simulink model "FCEvReferenceApplication"  (R2023a)
settings: Solver=ode23t  StartTime=0  StopTime=1435  RelTol=1e-3  EnableMultiTasking=on
libraries: autolibshared x1
settings Model: DataDictionary=VehicleConfig.sldd  ModifiedByFormat=The MathWorks, Inc.  SimulationMode=accelerator  PauseTimes=0  Creator=The MathWorks, Inc.  LastModifiedBy=The MathWorks, Inc.
settings SolverCC: MaxConsecutiveMinStep=12  ZeroCrossAlgorithm=Adaptive  AlgebraicLoopSolver=TrustRegion  AutoInsertRateTranBlk=on  DecoupledContinuousIntegration=on  MinimalZcImpactIntegration=on  MaxZcPerStep=1
settings DataIOCC: SaveOutput=off  DSMLogging=off  SaveTime=off  ReturnWorkspaceOutputs=off
settings OptimizationCC: ReuseModelBlockBuffer=off
settings DebuggingCC: UnderspecifiedInitializationDetection=Classic  MergeDetectMultiDrivingBlocksExec=none  IgnoredZcDiagnostic=none  UnconnectedInputMsg=warning  UnconnectedOutputMsg=warning  UnconnectedLineMsg=warning  ModelReferenceExtraNoncontSigs=none  PregeneratedLibrarySubsystemCodeDiagnostic=none  ArithmeticOperatorsInVariantConditions=warning
settings ModelReferenceCC: UpdateModelReferenceTargets=IfOutOfDate  EnableRefExpFcnMdlSchedulingChecks=on  ModelReferenceMinAlgLoopOccurrences=on  PropagateSignalLabelsOutOfModel=off
settings SFSimCC: SimUseLocalCustomCode=off
settings RTWCC: RTWUseLocalCustomCode=off  Toolchain=Microsoft Visual C++ 2022 v17.0 | CMake/nmake (64-bit Windows)  BuildConfiguration=Release  DLArmComputeVersion=19.05
settings CodeAppCC: StateflowObjectComments=on
settings GRTTargetCC: TargetLangStandard=C89/C90 (ANSI)
settings ConfigComp: CovMetricSettings=dsw  CovSaveCumulativeToWorkspaceVar=on  CovSaveSingleToWorkspaceVar=on  CovExternalEMLEnable=off

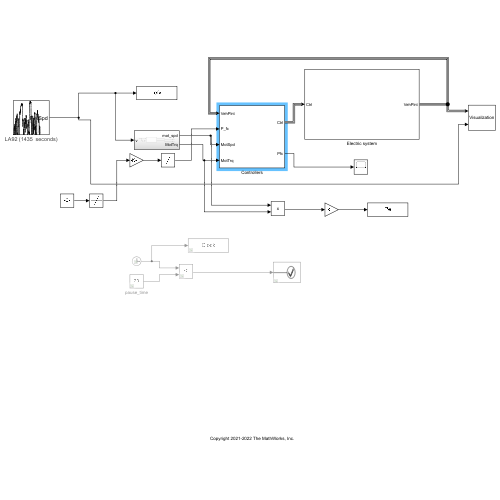
[thumbnail: Simulink's stored preview of the top-level diagram]
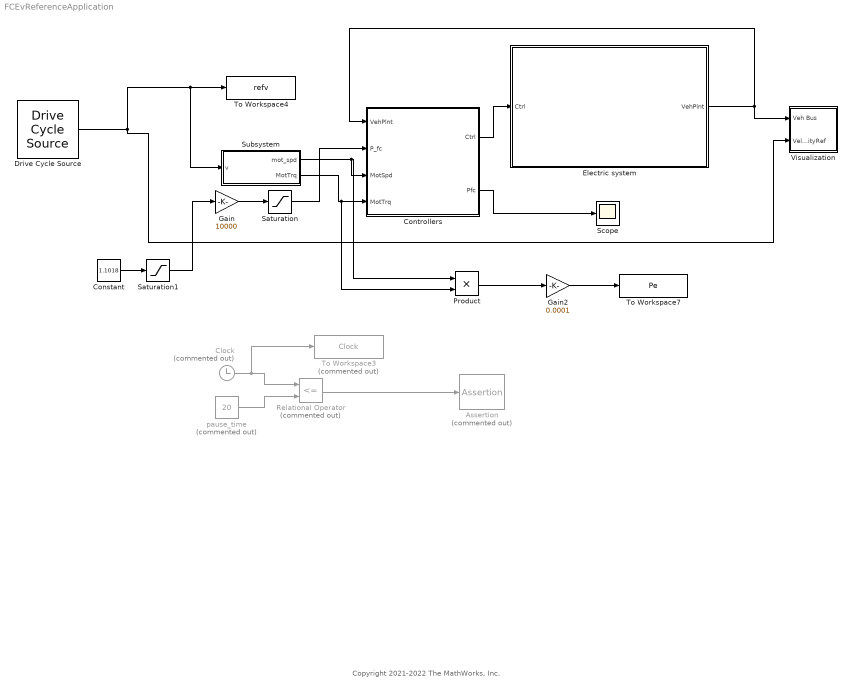
== system FCEvReferenceApplication ==
  note: Copyright 2021-2022 The MathWorks, Inc.
  Assertion : Assertion  Commented=on  AssertionFailFcn=set_param(bdroot, 'SimulationCommand', 'pause')  StopWhenAssertionFail=off
  Clock : Clock  Commented=on
  Constant : Constant  Value=1.1018
  Controllers : Subsystem
  Drive Cycle Source : autolibshared/Drive Cycle Source  cycleVar=LA92  fileVar=C:\Users\Leviathan\Desktop\WLTC工况.xlsx  tfinal="1435  seconds"  cycleRepeat=off  outAccPort=off  outGearPort=off  gearList=No gear data  t_wot1=1  xdot_woto=0  xdot_wot1=26.8  t_wot2=30  xdot_wot2=0  t_wotend=40  srcUnit=m/s  outUnit=m/s  srcAccUnit=m/s/s  outAccUnit=m/s^2  dt=0  aMode=1  faultOption=off  velBnd=2  velBndUnit=mph  inUnit=m/s  timeBnd=1  failOption=off  stopSim=off  maxFaultCnt=10  maxFaultTime=2  maxTotFaultTime=15  traceOption=off  dtTrace=1  traceWindow=10  lastDCname=LA92  lastOutUnit=mph  lastDT=0  lastTB=1  lastSB=2  forceCalcBound=off
  Electric system : Subsystem
  Gain : Gain  Gain=10000
  Gain2 : Gain  Gain=0.0001
  Product : Product
  Relational Operator : RelationalOperator  Commented=on  Operator=<=  OutDataTypeStr=boolean  RndMeth=Simplest  InputSameDT=off
  Saturation : Saturate  UpperLimit=inf  LowerLimit=200
  Saturation1 : Saturate  UpperLimit=35  LowerLimit=0
  Scope : Scope
  Subsystem : Subsystem
  To Workspace3 : ToWorkspace  Commented=on  VariableName=Clock  SampleTime=1
  To Workspace4 : ToWorkspace  VariableName=refv  SampleTime=1
  To Workspace7 : ToWorkspace  VariableName=Pe  SampleTime=1
  Visualization : Subsystem
      mask Display: disp(getString(message('autoblks:autoblkVehMask:visual')))
  pause_time : Constant  Commented=on  Value=20
  wires:
  Controllers/1(Ctrl) -> Electric system/1(Ctrl)
  Electric system/1(VehPlnt) -> Visualization/1(Veh Bus), Controllers/1(VehPlnt)
  Controllers/2(Pfc) -> Scope/1
  pause_time/1 -> Relational Operator/2
  Clock/1 -> To Workspace3/1, Relational Operator/1
  Relational Operator/1 -> Assertion/1
  Gain/1 -> Saturation/1
  Constant/1 -> Saturation1/1
  Saturation1/1 -> Gain/1
  Subsystem/1(mot_spd) -> Product/1, Controllers/3(MotSpd)
  Subsystem/2(MotTrq) -> Product/2, Controllers/4(MotTrq)
  Drive Cycle Source/1 -> Visualization/2(VelocityRef), Subsystem/1(v), To Workspace4/1
  Gain2/1 -> To Workspace7/1
  Product/1 -> Gain2/1
  Saturation/1 -> Controllers/2(P_fc)

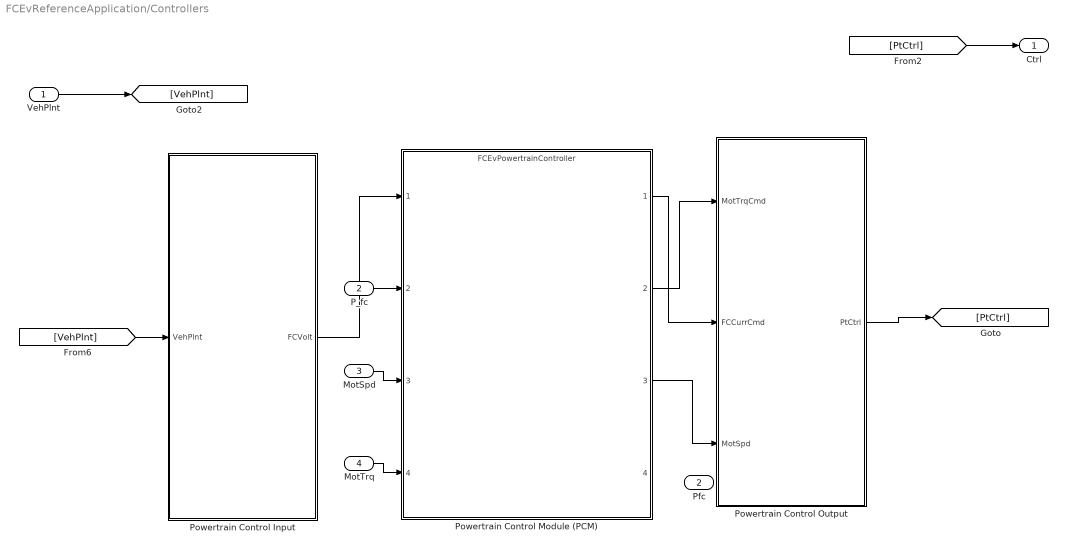
== system FCEvReferenceApplication/Controllers ==
  VehPlnt : Inport
  P_fc : Inport  Port=2
  MotSpd : Inport  Port=3
  MotTrq : Inport  Port=4
  Powertrain Control Input : Subsystem
  Powertrain Control Module (PCM) : ModelReference  ModelNameDialog=FCEvPowertrainController.slx  ModelReferenceVersion=6.39
  Powertrain Control Output : Subsystem
  Ctrl : Outport  VectorParamsAs1DForOutWhenUnconnected=off
  Pfc : Outport  Port=2
  wires:
  VehPlnt/1 -> [VehPlnt]
  [PtCtrl] -> Ctrl/1
  [VehPlnt] -> Powertrain Control Input/1(VehPlnt)
  Powertrain Control Output/1(PtCtrl) -> [PtCtrl]
  Powertrain Control Input/1(FCVolt) -> Powertrain Control Module (PCM)/1
  Powertrain Control Module (PCM)/1 -> Powertrain Control Output/2(FCCurrCmd)
  Powertrain Control Module (PCM)/3 -> Powertrain Control Output/3(MotSpd)
  MotTrq/1 -> Powertrain Control Module (PCM)/4
  MotSpd/1 -> Powertrain Control Module (PCM)/3
  Powertrain Control Module (PCM)/2 -> Powertrain Control Output/1(MotTrqCmd)
  P_fc/1 -> Powertrain Control Module (PCM)/2
  ? -> Pfc/1

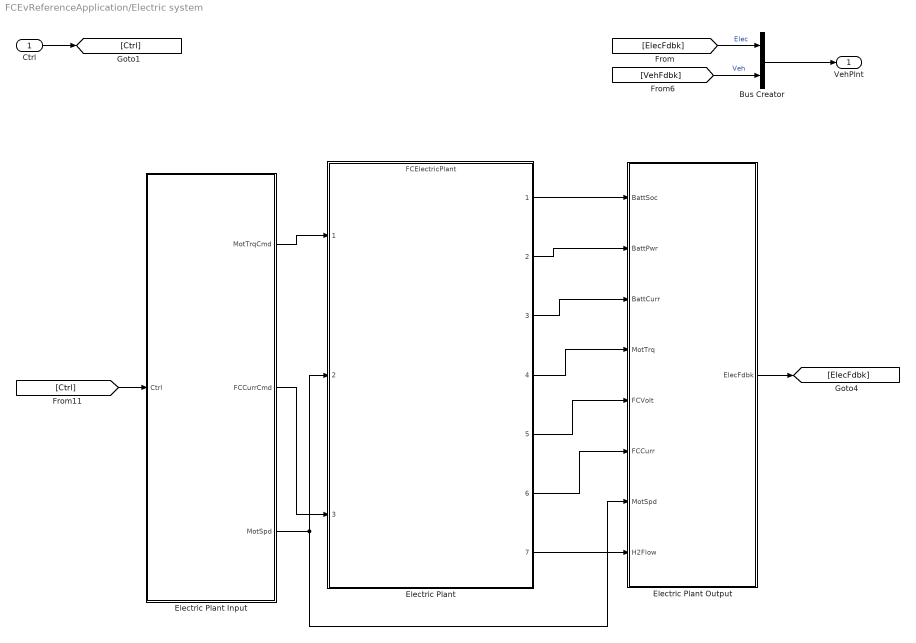
== system FCEvReferenceApplication/Electric system ==
  Ctrl : Inport
  Bus Creator : BusCreator  Inputs=2
  Electric Plant : ModelReference  ModelNameDialog=FCElectricPlant.slx  ModelReferenceVersion=6.24
  Electric Plant Input : Subsystem
  Electric Plant Output : Subsystem
  VehPlnt : Outport  VectorParamsAs1DForOutWhenUnconnected=off
  wires:
  Electric Plant/1 -> Electric Plant Output/1(BattSoc)
  Electric Plant/6 -> Electric Plant Output/6(FCCurr)
  Electric Plant/5 -> Electric Plant Output/5(FCVolt)
  Electric Plant/3 -> Electric Plant Output/3(BattCurr)
  Electric Plant/4 -> Electric Plant Output/4(MotTrq)
  Bus Creator/1 -> VehPlnt/1
  [ElecFdbk] -> Bus Creator/1  "Elec"
  Electric Plant Output/1(ElecFdbk) -> [ElecFdbk]
  Electric Plant Input/1(MotTrqCmd) -> Electric Plant/1
  Electric Plant/2 -> Electric Plant Output/2(BattPwr)
  [VehFdbk] -> Bus Creator/2  "Veh"
  [Ctrl] -> Electric Plant Input/1(Ctrl)
  Ctrl/1 -> [Ctrl]
  Electric Plant Input/2(FCCurrCmd) -> Electric Plant/3
  Electric Plant Input/3(MotSpd) -> Electric Plant Output/7(MotSpd), Electric Plant/2
  Electric Plant/7 -> Electric Plant Output/8(H2Flow)

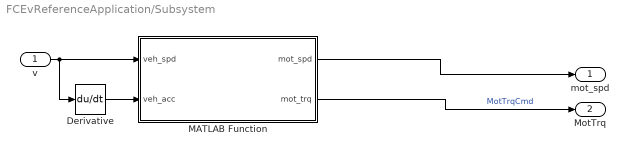
== system FCEvReferenceApplication/Subsystem ==
  v : Inport
  Derivative : Derivative
  MATLAB Function : MATLAB Function  TreatAsAtomicUnit=on
  mot_spd : Outport
  MotTrq : Outport  Port=2
  wires:
  v/1 -> Derivative/1, MATLAB Function/1(veh_spd)
  MATLAB Function/1(mot_spd) -> mot_spd/1
  MATLAB Function/2(mot_trq) -> MotTrq/1  "MotTrqCmd"
  Derivative/1 -> MATLAB Function/2(veh_acc)

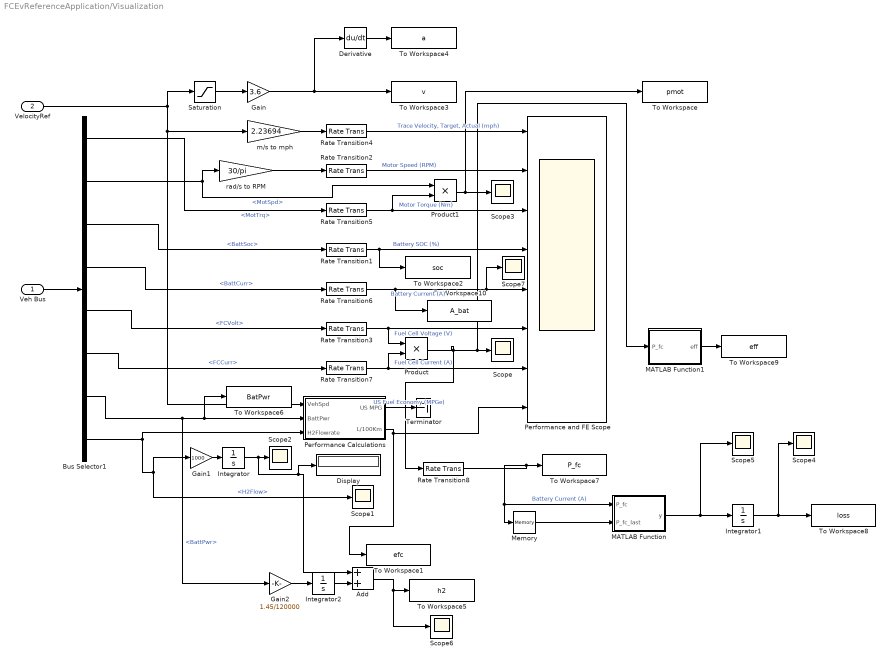
== system FCEvReferenceApplication/Visualization ==
  Veh Bus : Inport
  VelocityRef : Inport  Port=2
  Add : Sum
  Bus Selector1 : BusSelector  OutputSignals=Elec.MotTrq,Elec.MotSpd,Elec.BattSoc,Elec.BattCurr,Elec.FCVolt,Elec.FCCurr,Elec.BattPwr,Elec.H2Flow
  Derivative : Derivative
  Display : Display
  Gain : Gain  Gain=3.6
  Gain1 : Gain  Gain=1000
  Gain2 : Gain  Gain=1.45/120000
  Integrator : Integrator
  Integrator1 : Integrator
  Integrator2 : Integrator
  MATLAB Function : MATLAB Function  TreatAsAtomicUnit=on
  MATLAB Function1 : MATLAB Function  TreatAsAtomicUnit=on
  Memory : Memory  InheritSampleTime=on
  Performance Calculations : Subsystem
  Performance and FE Scope : Scope  NumInputPorts=8
  Product : Product
  Product1 : Product
  Rate Transition{1..2,4..6} (5 alike) : RateTransition  Deterministic=off
  Rate Transition3 : RateTransition  Deterministic=off  OutPortSampleTime=1
  Rate Transition7 : RateTransition  Deterministic=off  OutPortSampleTime=1
  Rate Transition8 : RateTransition  Deterministic=off  OutPortSampleTime=1
  Saturation : Saturate  UpperLimit=Inf  LowerLimit=0
  Scope{,1..7} (8 alike) : Scope
  Terminator : Terminator
  To Workspace : ToWorkspace  VariableName=pmot  SampleTime=1
  To Workspace1 : ToWorkspace  VariableName=efc  SampleTime=1
  To Workspace10 : ToWorkspace  VariableName=A_bat  SampleTime=1
  To Workspace2 : ToWorkspace  VariableName=soc  SampleTime=1
      settings: Save2DSignal=2-D array (concatenate along first dimension)
  To Workspace3 : ToWorkspace  VariableName=v  SampleTime=1
  To Workspace4 : ToWorkspace  VariableName=a  SampleTime=1
  To Workspace5 : ToWorkspace  VariableName=h2  SampleTime=1
  To Workspace6 : ToWorkspace  VariableName=BatPwr  SampleTime=1
      settings: Save2DSignal=2-D array (concatenate along first dimension)
  To Workspace7 : ToWorkspace  VariableName=P_fc  SampleTime=1
  To Workspace8 : ToWorkspace  VariableName=loss  SampleTime=1
  To Workspace9 : ToWorkspace  VariableName=eff  SampleTime=1
  m/s to mph : Gain  Gain=2.23694
  rad/s to RPM : Gain  Gain=30/pi
  wires:
  Veh Bus/1 -> Bus Selector1/1
  VelocityRef/1 -> Performance Calculations/1(VehSpd), m/s to mph/1, Saturation/1
  Performance Calculations/2(L/100Km) -> Performance and FE Scope/8, To Workspace1/1
  m/s to mph/1 -> Rate Transition4/1
  Bus Selector1/3 -> Rate Transition1/1  "<BattSoc>"
  Rate Transition1/1 -> To Workspace2/1, Performance and FE Scope/4  "Battery SOC (%)"
  Rate Transition2/1 -> Performance and FE Scope/2  "Motor Speed (RPM)"
  Rate Transition4/1 -> Performance and FE Scope/1  "Trace Velocity, Target, Actual (mph)"
  Bus Selector1/2 -> rad/s to RPM/1, Product1/1  "<MotSpd>"
  Bus Selector1/7 -> Gain2/1, Performance Calculations/2(BattPwr), To Workspace6/1  "<BattPwr>"
  rad/s to RPM/1 -> Rate Transition2/1
  Bus Selector1/1 -> Rate Transition5/1  "<MotTrq>"
  Rate Transition5/1 -> Product1/2, Performance and FE Scope/3  "Motor Torque (Nm)"
  Rate Transition6/1 -> To Workspace10/1, Scope7/1, Performance and FE Scope/5  "Battery Current (A)"
  Bus Selector1/4 -> Rate Transition6/1  "<BattCurr>"
  Bus Selector1/8 -> Performance Calculations/3(H2Flowrate), Scope1/1, Gain1/1  "<H2Flow>"
  Bus Selector1/6 -> Rate Transition7/1  "<FCCurr>"
  Rate Transition7/1 -> Performance and FE Scope/7, Product/2  "Fuel Cell Current (A)"
  Bus Selector1/5 -> Rate Transition3/1  "<FCVolt>"
  Rate Transition3/1 -> Performance and FE Scope/6, Product/1  "Fuel Cell Voltage (V)"
  Product/1 -> Rate Transition8/1, MATLAB Function1/1(P_fc), Scope/1
  Saturation/1 -> Gain/1
  Gain/1 -> Derivative/1, To Workspace3/1
  Derivative/1 -> To Workspace4/1
  Integrator/1 -> Add/1, Display/1, Scope2/1
  Gain1/1 -> Integrator/1
  Performance Calculations/1(US MPG) -> Terminator/1  "US Fuel Economy (MPGe)"
  Product1/1 -> To Workspace/1, Scope3/1
  Memory/1 -> MATLAB Function/2(P_fc_last)
  MATLAB Function/1(y) -> Scope5/1, Integrator1/1
  Integrator1/1 -> Scope4/1, To Workspace8/1
  Gain2/1 -> Integrator2/1
  Add/1 -> Scope6/1, To Workspace5/1
  Integrator2/1 -> Add/2
  MATLAB Function1/1(eff) -> To Workspace9/1
  Rate Transition8/1 -> Memory/1, MATLAB Function/1(P_fc), To Workspace7/1  "Battery Current (A)"

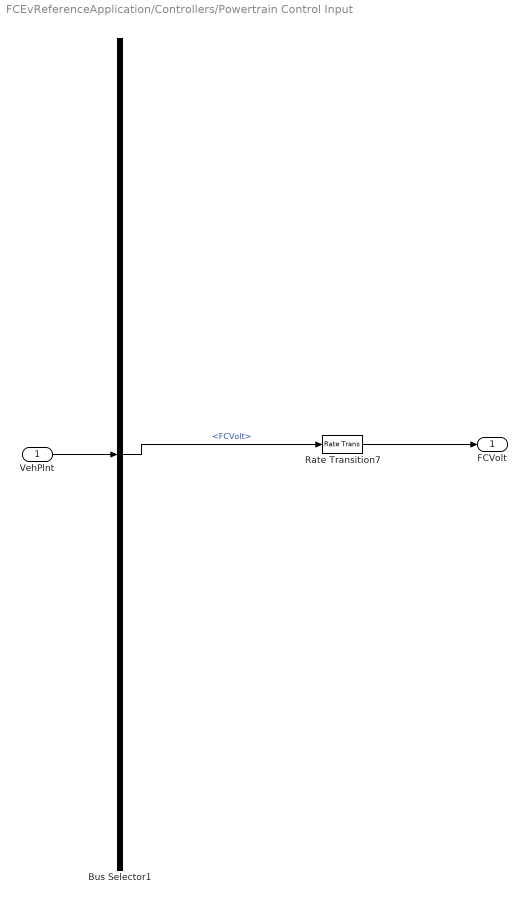
== system FCEvReferenceApplication/Controllers/Powertrain Control Input ==
  VehPlnt : Inport
  Bus Selector1 : BusSelector  OutputSignals=Elec.FCVolt
  Rate Transition7 : RateTransition  Deterministic=off
  FCVolt : Outport  VectorParamsAs1DForOutWhenUnconnected=off
  wires:
  VehPlnt/1 -> Bus Selector1/1
  Rate Transition7/1 -> FCVolt/1
  Bus Selector1/1 -> Rate Transition7/1  "<FCVolt>"

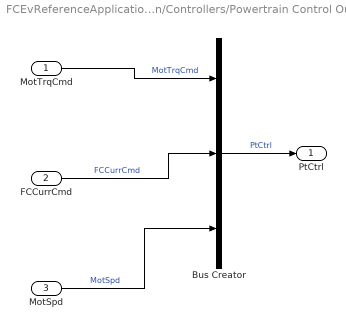
== system FCEvReferenceApplication/Controllers/Powertrain Control Output ==
  MotTrqCmd : Inport
  FCCurrCmd : Inport  Port=2
  MotSpd : Inport  Port=3
  Bus Creator : BusCreator  Inputs=3
  PtCtrl : Outport  VectorParamsAs1DForOutWhenUnconnected=off
  wires:
  Bus Creator/1 -> PtCtrl/1  "PtCtrl"
  MotTrqCmd/1 -> Bus Creator/1  "MotTrqCmd"
  FCCurrCmd/1 -> Bus Creator/2  "FCCurrCmd"
  MotSpd/1 -> Bus Creator/3  "MotSpd"

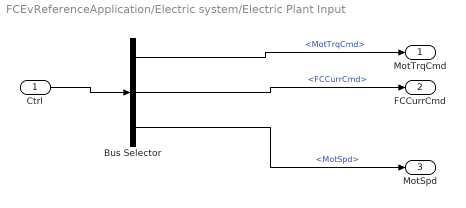
== system FCEvReferenceApplication/Electric system/Electric Plant Input ==
  Ctrl : Inport
  Bus Selector : BusSelector  OutputSignals=MotTrqCmd,FCCurrCmd,MotSpd
  MotTrqCmd : Outport  VectorParamsAs1DForOutWhenUnconnected=off
  FCCurrCmd : Outport  Port=2  VectorParamsAs1DForOutWhenUnconnected=off
  MotSpd : Outport  Port=3  VectorParamsAs1DForOutWhenUnconnected=off
  wires:
  Ctrl/1 -> Bus Selector/1
  Bus Selector/1 -> MotTrqCmd/1  "<MotTrqCmd>"
  Bus Selector/2 -> FCCurrCmd/1  "<FCCurrCmd>"
  Bus Selector/3 -> MotSpd/1  "<MotSpd>"

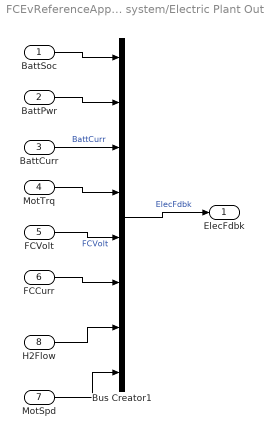
== system FCEvReferenceApplication/Electric system/Electric Plant Output ==
  BattSoc : Inport
  BattPwr : Inport  Port=2
  BattCurr : Inport  Port=3
  MotTrq : Inport  Port=4
  FCVolt : Inport  Port=5
  FCCurr : Inport  Port=6
  MotSpd : Inport  Port=7
  H2Flow : Inport  Port=8
  Bus Creator1 : BusCreator  Inputs=8
  ElecFdbk : Outport  VectorParamsAs1DForOutWhenUnconnected=off
  wires:
  Bus Creator1/1 -> ElecFdbk/1  "ElecFdbk"
  BattPwr/1 -> Bus Creator1/2
  BattSoc/1 -> Bus Creator1/1
  BattCurr/1 -> Bus Creator1/3  "BattCurr"
  MotTrq/1 -> Bus Creator1/4
  FCVolt/1 -> Bus Creator1/5  "FCVolt"
  FCCurr/1 -> Bus Creator1/6
  H2Flow/1 -> Bus Creator1/7
  MotSpd/1 -> Bus Creator1/8

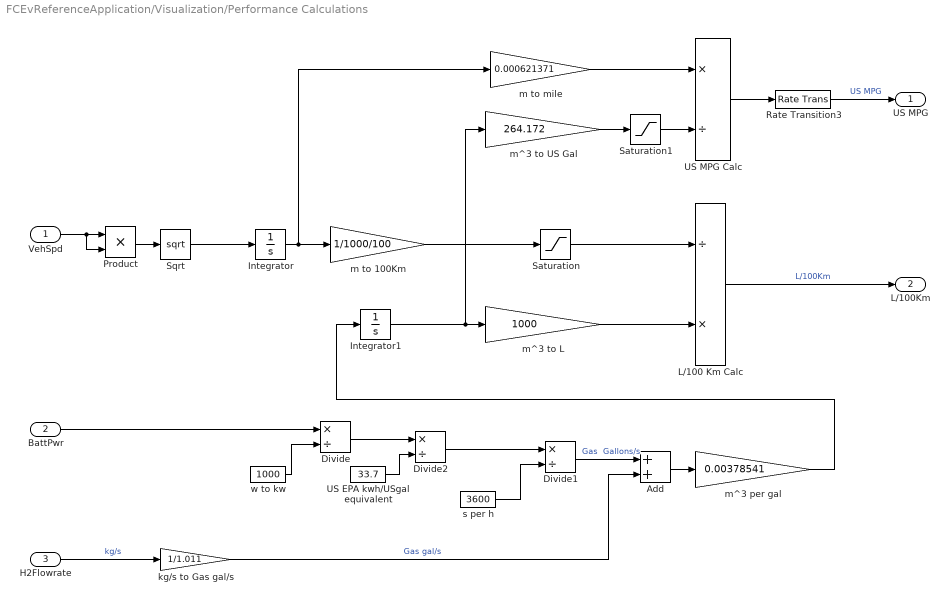
== system FCEvReferenceApplication/Visualization/Performance Calculations ==
  VehSpd : Inport
  BattPwr : Inport  Port=2
  H2Flowrate : Inport  Port=3
  Add : Sum
  Divide : Product  Inputs=*/
  Divide1 : Product  Inputs=*/
  Divide2 : Product  Inputs=*/
  Integrator : Integrator
  Integrator1 : Integrator
  L/100 Km Calc : Product  Inputs=/*
  Product : Product
  Rate Transition3 : RateTransition  Deterministic=off
  Saturation : Saturate  UpperLimit=Inf  LowerLimit=0.001
  Saturation1 : Saturate  UpperLimit=Inf  LowerLimit=1e-3
  Sqrt : Sqrt
  US EPA kwh/USgal equivalent : Constant  Value=33.7
  US MPG Calc : Product  Inputs=*/
  kg/s to Gas gal/s : Gain  Gain=1/1.011
  m to 100Km : Gain  Gain=1/1000/100
  m to mile : Gain  Gain=0.000621371
  m^3 per gal : Gain  Gain=0.00378541
  m^3 to L : Gain  Gain=1000
  m^3 to US Gal : Gain  Gain=264.172
  s per h : Constant  Value=3600
  w to kw : Constant  Value=1000
  US MPG : Outport  VectorParamsAs1DForOutWhenUnconnected=off
  L/100Km : Outport  Port=2  VectorParamsAs1DForOutWhenUnconnected=off
  wires:
  m^3 to US Gal/1 -> Saturation1/1
  m^3 to L/1 -> L/100 Km Calc/2
  Integrator/1 -> m to mile/1, m to 100Km/1
  m to mile/1 -> US MPG Calc/1
  Integrator1/1 -> m^3 to US Gal/1, m^3 to L/1
  Saturation/1 -> L/100 Km Calc/1
  m to 100Km/1 -> Saturation/1
  L/100 Km Calc/1 -> L/100Km/1  "L/100Km"
  US MPG Calc/1 -> Rate Transition3/1
  Saturation1/1 -> US MPG Calc/2
  Rate Transition3/1 -> US MPG/1  "US MPG"
  w to kw/1 -> Divide/2
  Divide/1 -> Divide2/1
  Divide2/1 -> Divide1/1
  s per h/1 -> Divide1/2
  Divide1/1 -> Add/1  "Gas  Gallons/s"
  US EPA kwh/USgal equivalent/1 -> Divide2/2
  BattPwr/1 -> Divide/1
  Sqrt/1 -> Integrator/1
  Product/1 -> Sqrt/1
  VehSpd/1 -> Product/2, Product/1
  m^3 per gal/1 -> Integrator1/1
  H2Flowrate/1 -> kg/s to Gas gal/s/1  "kg/s"
  kg/s to Gas gal/s/1 -> Add/2  "Gas gal/s"
  Add/1 -> m^3 per gal/1

== matlab function FCEvReferenceApplication/Visualization/MATLAB Function ==
  data: P_fc input; y output; P_fc_last input
function y = fcn(P_fc, P_fc_last)
u=0;
if((P_fc==0&&P_fc_last>0))
    u=u+0.00196;
end
if(P_fc>0&&P_fc<=7000)
    u=u+0.00126/3600;
end
if(abs(P_fc-P_fc_last)>12000) 
    u=u+0.00005963;
end
if(P_fc>63000)
    u=u+0.00147/3600;
end

y = u;

== matlab function FCEvReferenceApplication/Visualization/MATLAB Function1 ==
  data: P_fc input; eff output
function eff = fcn(P_fc)
fc_pwr_map = [0	1072.90229853803	1216.85650798951	1359.59851460102	1501.35017957354	1642.27676444055	1782.53778025993	1922.24351589635	2061.42626733138	2200.07476094921	2338.17130192102	2475.70683694821	2612.68288708918	2749.10918467404	2885.00072139605	3020.37535249597	3155.25212611030	3289.65020692397	3423.58823588020	3557.08391827318	3690.15380512072	3823.07558594165	3955.85245344655	4088.37561795968	4220.61488906977	4352.56406363307	4484.22506138967	4615.60845349907	4746.72537153320	4877.58617634250	5008.20101841421	5138.57910701179	5268.72893779909	5398.65843210451	5528.37491810699	5657.88512121010	5787.19531790160	5916.31126144911	6045.23838229580	6173.98170377466	6302.54592100281	6430.93523576898	6559.15407939906	6686.36322605221	6812.91227829557	6939.23197241272	7065.32770458568	7191.20233240135	7316.85868136767	7442.29946015133	7567.52735310215	7692.54476785426	7817.35414262247	7941.95794027495	8066.35839410929	8190.55721576634	8314.55761866446	8438.36117790742	8561.96941744725	8685.38463779521	8808.60863685525	8931.64323689573	9054.49014325740	9177.15069874731	9299.62695433075	9421.92021588226	9544.03195449078	9665.96362107524	9787.71705237388	9909.29339377050	10030.6937637603	10151.9199164870	10272.9726013835	10393.8537048637	10514.5636761990	10635.1045530165	10755.4772713985	10875.6826157159	10995.7216879776	11115.5959476105	11235.3059832979	11354.8530825862	11474.2382729129	11593.4622572804	11712.5261226507	11831.4307634265	11950.1772445910	12068.7664326711	12187.1991631663	12305.4762984413	12423.5986606479	12541.5671462540	12659.3824194685	12777.0451010561	12894.5559678070	13011.9203853400	13129.1509406938	13246.2534270434	13363.2291458499	13480.0764252504	13596.7929126851	13713.3756818561	13829.8227998316	13946.1318121346	14062.3022020181	14178.3328702196	14294.2229916514	14409.9724360912	14525.5811090914	14641.0491037678	14756.3766437677	14871.5640268236	14986.6116165973	15101.5198142293	15216.2890283615	15330.9196985154	15445.4122669574	15559.7671786892	15673.9848782481	15788.0658123241	15902.0104005133	16015.8190981300	16129.4923319684	16243.0305028681	16356.4340315659	16469.7033383789	16582.8388327729	16695.8408921659	16808.7099143940	16921.4462843248	17034.0503807289	17146.5225766003	17258.8632395181	17371.0727307757	17483.1514069888	17595.0996192849	17706.9177135773	17818.6060306982	17930.1649065130	18041.5946720314	18152.8956534897	18264.0681724165	18375.1125459202	18486.0290866848	18596.8181030627	18707.4798991736	18818.0147750123	18928.4230265502	19038.7049458338	19148.8608210861	19258.8909368034	19368.7955738538	19478.5750095701	19588.2295178478	19697.7593692369	19807.1648310362	19916.4461673844	20025.6036393511	20134.6375050283	20243.5480196198	20352.3354355281	20461.0000024441	20569.5419583178	20677.9613366887	20786.2582763735	20894.4329891170	21002.4856857775	21110.4165737466	21218.2258576406	21325.9137386505	21433.4804149482	21540.9260816950	21648.2509310959	21755.4551524525	21862.5389322177	21969.5024540466	22076.3458988475	22183.0694448317	22289.6732675625	22396.1575400017	22502.5224325584	22608.7681131334	22714.8947471644	22820.9024976699	22926.7915255296	23032.5619885719	23138.2140430316	23243.7478426889	23349.1635390930	23454.4612816159	23559.6412174922	23664.7034918522	23769.6482477691	23874.4756262756	23979.1857662239	24083.7788051244	24188.2548782964	24292.6141177574	24396.8566560881	24500.9826225012	24604.9921447184	24708.8853487057	24812.6623586889	24916.3232971743	25019.8682849774	25123.2974412481	25226.6108834969	25329.8087283243	25432.8910951689	25535.8580953686	25638.7098392918	25741.4464360553	25844.0679934139	25946.5746177226	26048.9664139350	26151.2434856103	26253.4059349319	26355.4538627218	26457.3873684589	26559.2065502960	26660.9115050783	26762.5023283583	26863.9791144160	26965.3419562732	27066.5909457112	27167.7261732871	27268.7477283497	27369.6556988230	27470.4501724288	27571.1312344540	27671.6989694970	27772.1534609557	27872.4947914538	27972.7230415141	28072.8382934268	28172.8406249958	28272.7301143478	28372.5068379005	28472.1708730543	28571.7222948795	28671.1611756256	28770.4875900029	28869.7016088879	28968.8033038351	29067.7927456532	29166.6700009573	29265.4351410368	29364.0882311638	29462.6293378617	29561.0585278605	29659.3758642078	29757.5814127060	29855.6752333201	29953.6573896758	30051.5279441430	30149.2869541207	30246.9344811739	30344.4705812342	30441.8953166342	30539.2087409038	30636.4109109773	30733.5018838060	30830.4817119931	30927.3504493040	31024.1081505306	31120.7548677213	31217.2906517159	31313.7155540694	31410.0296252259	31506.2329140046	31602.3254692233	31698.3073383118	31794.1785706267	31889.9392114267	31985.5893083038	32081.1289051060	32176.5580393561	32271.8767731494	32367.0851314515	32462.1831750984	32557.1709336173	32652.0484365215	32746.8157560826	32841.4729132667	32936.0199457077	33030.4568954387	33124.7838017361	33219.0007025099	33313.1076350149	33407.1046359050	33500.9917412524	33594.7689865564	33688.4364067506	33781.9940362081	33875.4419087470	33968.7800576358	34062.0085155983	34155.1273148186	34248.1364869463	34341.0360631010	34433.8260738774	34526.5065493500	34619.0775190775	34711.5390121075	34803.8910569812	34896.1336817376	34988.2669139178	35080.2907805694	35172.2053082509	35264.0105230356	35355.7064505156	35447.2931158062	35538.7705435497	35630.1387579189	35721.3977826219	35812.5476409047	35903.5883555560	35994.5199489099	36085.3424428503	36176.0558588141	36266.6602177945	36357.1555403447	36447.5418465812	36537.8191561868	36627.9874884137	36718.0468620924	36807.9972956521	36897.8388064232	36987.5714148569	37077.1951316354	37166.7099815673	37256.1159764884	37345.4131326168	37434.6014652443	37523.6809882887	37612.6517205548	37701.5136755881	37790.2668617476	37878.9113010630	37967.4469998307	38055.8739719661	38144.1922344474	38232.4017919209	38320.5026639513	38408.4948569091	38496.3783818645	38584.1532498217	38671.8194716138	38759.3770554219	38846.8260171863	38934.1663552337	39021.3980889073	39108.5212184187	39195.5357542094	39282.4417050597	39369.2390763022	39455.9278801580	39542.5081155022	39628.9797955120	39715.3429183853	39801.5975009052	39887.7435340865	39973.7810346339	40059.7100040410	40145.5304444445	40231.2423595321	40316.8457548053	40402.3406326924	40487.7269976791	40573.0048462650	40658.1741866390	40743.2350213062	40828.1873485090	40913.0311681843	40997.7664859524	41082.3933016231	41166.9116131656	41251.3214203934	41335.6227243448	41419.8155252494	41503.8998200881	41587.8756099395	41671.7428900774	41755.5016609092	41839.1519192180	41922.6936633144	42006.1268884477	42089.4515951743	42172.6677811454	42255.7754342086	42338.7745550390	42421.6651440621	42504.4471861039	42587.1206909397	42669.6856363061	42752.1420353471	42834.4898665379	42916.7291298686	42998.8598185426	43080.8819258193	43162.7954446843	43244.6003678324	43326.2966876657	43407.8843962929	43489.3634855305	43570.7339469027	43651.9957716425	43733.1489506919	43814.1934747025	43895.1293340358	43975.9565187637	44056.6750186693	44137.2848232468	44217.7859217018	44298.1783029480	44378.4619556135	44458.6368680409	44538.7030282862	44618.6604241183	44698.5090430196	44778.2488721863	44857.8798985287	44937.4021086708	45016.8154889513	45096.1200254229	45175.3157038531	45254.4025097240	45333.3804293648	45412.2494457548	45491.0095440173	45569.6607087645	45648.2029240795	45726.6361737368	45804.9604412226	45883.1757097371	45961.2819621953	46039.2791812265	46117.1673491744	46194.9464480970	46272.6164597663	46350.1773656683	46427.6291470025	46504.9717846821	46582.2052593333	46659.3295512954	46736.3446406205	46813.2505070733	46890.0471301314	46966.7344889853	47043.3125625399	47119.7813294180	47196.1407679646	47272.3908562388	47348.5315718991	47424.5628919053	47500.4847934634	47576.2972549972	47652.0002531537	47727.5937613336	47803.0777564183	47878.4522148992	47953.7171159154	48028.8724262885	48103.9181292910	48178.8541917212	48253.6805964530	48328.3973045069	48403.0043050447	48477.5015583215	48551.8890453300	48626.1667370135	48700.3346048106	48774.3926196093	48848.3407623172	48922.1789814024	48995.9072845435	49069.5255982399	49143.0339365833	49216.4322370277	49289.7204867359	49362.8986515809	49435.9666961282	49508.9245998386	49581.7723185915	49654.5098288567	49727.1371042730	49799.6540868415	49872.0607851764	49944.3571308817	50016.5431082795	50088.6186744496	50160.5838015512	50232.4384609531	50304.1826046876	50375.8162067835	50447.3392281407	50518.7516349589	50590.0533948548	50661.2444656159	50732.3248124525	50803.2944073296	50874.1531948375	50944.9011540082	51015.5382432025	51086.0644147217	51156.4796473332	51226.7838808710	51296.9770955175	51367.0592431206	51437.0302818589	51506.8901774298	51576.6388799449	51646.2763573015	51715.8025731417	51785.2174650111	51854.5210055884	51923.7131527021	51992.7938689932	52061.7630989072	52130.6207991010	52199.3669339624	52268.0014530667	52336.5243179310	52404.9354744994	52473.2348900323	52541.4225083641	52609.4982854867	52677.4621764791	52745.3141330789	52813.0541096260	52880.6820566070	52948.1979278393	53015.6016716701	53082.8932421026	53150.0725887989	53217.1396620389	53284.0944116785	53350.9367871610	53417.6667375153	53484.2842113533	53550.7891568670	53617.1815218258	53683.4612535738	53749.6282990271	53815.6826046705	53881.6241165549	53947.4527802944	54013.1685410629	54078.7713435918	54144.2611321661	54209.6378506218	54274.9014423426	54340.0518502567	54405.0890168336	54470.0128840807	54534.8233935403	54599.5204862857	54664.1041029182	54728.5741835635	54792.9306678681	54857.1734949960	54921.3026036249	54985.3179319426	55049.2194176433	55113.0069979237	55176.6806094796	55240.2401885018	55303.6856706721	55367.0169911595	55430.2340846163	55493.3368851739	55556.3253264388	55619.1993414881	55681.9588628840	55744.6038224849	55807.1341520943	55869.5497823677	55931.8506436675	55994.0366658645	56056.1077782172	56118.0639094558	56179.9049875703	56241.6309403242	56303.2416943561	56364.7371764158	56426.1173119189	56487.3820264036	56548.5312444664	56609.5648898660	56670.4828860264	56731.2851559164	56791.9716216419	56852.5422043816	56912.9968254495	56973.3354050804	57033.5578629035	57093.6641178409	57153.6540878110	57213.5276913436	57273.2848446148	57332.9254645268	57392.4494664283	57451.8567654253	57511.1472758165	57570.3209107836	57629.3775837550	57688.3172068679	57747.1396914427	57805.8449479429	57864.4328867924	57922.9034173309	57981.2564477330	58039.4918857200	58097.6096389392	58155.6096134410	58213.4917142579	58271.2558463159	58328.9019139457	58386.4298199063	58443.8394666767	58501.1307554980	58558.3035876832	58615.3578627975	58672.2934797479	58729.1103370604	58785.8083316889	58842.3873605489	58898.8473190376	58955.1881021339	59011.4096034135	59067.5117164890	59123.4943322215	59179.3573435102	59235.1006393120	59290.7241093397	59346.2276420551	59401.6111248477	59456.8744441731	59512.0174863190	59567.0401317307	59621.9422697798	59676.7237802235	59731.3845451023	59785.9244468340	59840.3433582453	59894.6411652363	59948.8177411356	60002.8729636412	60056.8067076956	60110.6188467521	60164.3092554611	60217.8778027339	60271.3243627439	60324.6488034608	60377.8509938007	60430.9308007142	60483.8880910079	60536.7227289302	60589.4345784351	60642.0235021753	60694.4893616082	60746.8320168325	60799.0513260745	60851.1471476163	60903.1193374577	60954.9677506127	61006.6922401799	61058.2926585934	61109.7688575484	61161.1206855611	61212.3479915575	61263.4506223603	61314.4284226054	61365.2812368930	61416.0089075800	61466.6112756196	61517.0881805867	61567.4394605268	61617.6649519638	61667.7644898832	61717.7379077134	61767.5850373068	61817.3057089203	61866.8997511955	61916.3669911390	61965.7072541019	62014.9203637592	62064.0061420887	62112.9644093501	62161.7949840629	62210.4976829843	62259.0723210874	62307.5187115379	62355.8366656712	62404.0259929691	62452.0865010355	62500.0179955724	62547.8202803548	62595.4931572065	62643.0364259735	62690.4498844986	62737.7333285953	62784.8865520200	62831.9093464457	62878.8015014336	62925.5628044051	62972.1930406132	63018.6919931127	63065.0594427313	63111.2951680388	63157.3989453162	63203.3705485250	63249.2097492746	63294.9163167906	63340.4900178811	63385.9306169038	63431.2378757311	63476.4115537161	63521.4514076564	63566.3571917586	63611.1286576015	63655.7655540985	63700.2676274597	63744.6346211533	63788.8662758659	63832.9623294017	63876.9225170083	63920.7465704918	63964.4342189967	64007.9851889318	64051.3992032620	64094.6759821399	64137.8152422858	64180.8166976555	64223.6800586268	64266.4050326508	64308.9913235024	64351.4386318984	64393.7466549305	64435.9150862230	64477.9436159502	64519.8319319600	64561.5797173159	64603.1866478138	64644.6524010390	64685.9766488327	64727.1590591639	64768.1992957834	64809.0970188021	64849.8518840751	64890.4635433415	64930.9316438512	64971.2558297917	65011.4357393790	65051.4710080515	65091.3612650843	65131.1061367211	65170.7052434858	65210.1582020590	65249.4646239071	65288.6241156865	65327.6362791855	65366.5007113014	65405.2170038499	65443.7847430430	65482.2035104489	65520.4728818225	65558.5924274810	65596.5617125532	65634.3802961008	65672.0477319530	65709.5635672208	65746.9273444042	65784.1385984545	65821.1968593570	65858.1016499691	65894.8524875079	65931.4488822028	65967.8903379624	66004.1763517742	66040.3064139208	66076.2800074138	66112.0966083498	66147.7556858243	66183.2567013246	66218.5991086662	66253.7823539134	66288.8058760151	66323.6691051775	66358.3714640867	66392.9123671443	66427.2912193468	66461.5074186728	66495.5603530591	66529.4494024164	66563.1739368014	66596.7333174948	66630.1268961806	66663.3540150095	66696.4140059508	66729.3061910641	66762.0298825775	66794.5843816671	66826.9689795162	66859.1829663590	66891.2256032367	66923.0961449824	66954.7938367268	66986.3179128755	67017.6675949848	67048.8420924543	67079.8406027022	67110.6623093500	67141.3063832761	67171.7719821018	67202.0582492126	67232.1643144445	67262.0892931227	67291.8322854742	67321.3923773578	67350.7686379485	67379.9601230523	67408.9658712096	67437.7849034564	67466.4162255734	67494.8588251607	67523.1116723683	67551.1737487394	67579.0439959890	67606.7213172247	67634.2045993279	67661.4927125476	67688.5845096822	67715.4788225131	67742.1744638973	67768.6702238397	67794.9648721623	67821.0571541097	67846.9457947647	67872.6294970368	67898.1069201626	67923.3766982282	67948.4374909032	67973.2876939512	67997.9248486770	68022.3476683417	68046.5550375355	68070.5456794069	68094.3181973697	68117.8711072052	68141.2028571178	68164.3118400227	68187.1964009204	68209.8548457072	68232.2854260588	68254.4863647174	68276.4558419554	68298.1919971099	68319.6929284766	68340.9566925214	68361.9813028676	68382.7647291613	68403.3048958411	68423.5996808309	68443.6469141619	68463.4443765294	68482.9897977855	68502.2808553696	68521.3151726721	68540.0903173335	68558.6037994728	68576.8530698450	68594.8355179227	68612.5484698995	68629.9891866101	68647.1548613651	68664.0426176931	68680.6495069890	68696.9725060610	68713.0085145720	68728.7543523701	68744.2067567026	68759.3623793057	68774.2177833657	68788.7694403428	68803.0137266508	68816.9469201842	68830.5651966857	68843.8646259429	68856.8411678065	68869.4906680184	68881.8088538404	68893.7913294688	68905.4335712553	68916.7309228623	68927.6785892043	68938.2716316629	68948.5049619892	68958.3733361499	68967.8713478478	68976.9934217079	68985.7338061003	68994.0865655772	69002.0455728990	69009.6045006213	69016.7568122140	69023.4957526819	69029.8143386501	69035.7053478802	69041.1613081755	69046.1744856325	69050.7368721919	69054.8401724385	69058.4757895946	69061.6348106466	69064.3079905404	69066.4857353740	69068.1580845099	69069.3146915234	69069.9448038933];
fc_eff_map = [0,	0.0278400528805473,	0.0982906391716858,	0.157789972087247,	0.208132235656687,	0.25091608864214,	0.287498055227787,	0.318979771266055,	0.346234828949267,	0.369961540910764,	0.390726515650271,	0.408993528411966,	0.42514382270494,	0.439491697164595,	0.45229700340828,	0.463775304000599,	0.474106128528229,	0.483439656893662,	0.491902215672189,	0.499600252571651,	0.506624184390766,	0.513101492895802,	0.519089823117714,	0.524620832278904,	0.529734985976314,	0.534471502679754,	0.538866021157019,	0.542951220882311,	0.546756036735203,	0.550305992096206,	0.553623752650472,	0.556729408571065,	0.559640841856475,	0.562374027497895,	0.56494326863709,	0.56736139866799,	0.569639974843967,	0.571789417488508,	0.573819162424791,	0.575737760743992,	0.577552983690564,	0.579271887117059,	0.580900964115041,	0.582358701423231,	0.583689191665366,	0.584944117530814,	0.586129033190926,	0.587248043272116,	0.588304999920716,	0.58930349413612,	0.590246876291348,	0.591138247185975,	0.591980503501378,	0.592776350688026,	0.593528297116033,	0.594238643346594,	0.594909667742709,	0.59554337004163,	0.596141621237337,	0.596706239236019,	0.597238892099624,	0.59774115062193,	0.598214484202633,	0.598660250000502,	0.599079780087056,	0.599474277019187,	0.599844888433151,	0.600192698024747,	0.60051875753316,	0.600824014752205,	0.601109366685412,	0.601375705648266,	0.601623812069673,	0.601854500527312,	0.602068453059022,	0.602266418735392,	0.60244904064063,	0.602616921974096,	0.602770656387416,	0.602910831242445,	0.603037954581419,	0.603152552262205,	0.603255111260344,	0.603346077818779,	0.60342590024172,	0.603494996356331,	0.603553775210872,	0.603602617275577,	0.603641885424689,	0.603671928475437,	0.603693078626625,	0.603705658336486,	0.603709964639825,	0.603706280541948,	0.603694883957715,	0.603575246282696,	0.603297126990593,	0.602915915016392,	0.602468098986328,	0.601977666109334,	0.601460398100054,	0.600926643336893,	0.600383222577884,	0.599834565552922,	0.599283629035156,	0.598732306377516,	0.598181818808023,	0.597632966913659,	0.597086253317952,	0.596541991403591,	0.596000369985115,	0.595461495312291,	0.59492542021259,	0.594392162362563,	0.59386171592901,	0.59333406114544,	0.592809168750835,	0.592287003733655,	0.591767527662752,	0.591250700417129,	0.590736480030705,	0.590224825997931,	0.589715697032318,	0.589209051502891,	0.588704849465852,	0.588203051924373,	0.587703620459535,	0.587206516457527,	0.586711703168571,	0.586219144386927,	0.585728804708844,	0.585240649526643,	0.584754645020801,	0.584270758104413,	0.583788956464415,	0.583309208509616,	0.582831483339747,	0.582355750727344,	0.581881981101552,	0.581410145531443,	0.580940215708067,	0.580472163928757,	0.580005963081108,	0.579541586631373,	0.579079008603918,	0.578618203566869,	0.57815914661829,	0.577701813372313,	0.577246179945763,	0.576792222945343,	0.576339919455106,	0.575889247024481,	0.575440183656639,	0.574992707797263,	0.574546798323755,	0.574102434534807,	0.573659596140267,	0.573218263251412,	0.572778416371554,	0.572340036386919,	0.57190310455787,	0.571467602510362,	0.571033511947793,	0.570600808804535,	0.570169472768417,	0.569739486172811,	0.569310831815323,	0.568883492504403,	0.568457451778427,	0.568032693178543,	0.567609200599572,	0.567186958213105,	0.566765950461305,	0.566346162050887,	0.565927577947267,	0.565510183368883,	0.565093963781681,	0.564678904893739,	0.564264992650052,	0.563852213227451,	0.563440553029652,	0.563029998682453,	0.562620537029045,	0.562212155125449,	0.561804840242485,	0.561398579835682,	0.560993361579331,	0.560589173338004,	0.560186003167531,	0.559783839311518,	0.559382670197576,	0.558982484433581,	0.558583270804178,	0.558185018251901,	0.557787716081166,	0.55739135033016,	0.556995918748071,	0.556601404064817,	0.556207797178349,	0.555815088579881,	0.555423268346487,	0.555032326703483,	0.554642254021265,	0.554253040812402,	0.553864677728874,	0.55347715555942,	0.553090465226951,	0.55270459780263,	0.552319544591826,	0.551935296870758,	0.551551846053856,	0.551169183683822,	0.550787301426295,	0.550406191066253,	0.550025844505297,	0.549646253759268,	0.549267410956042,	0.548889308333408,	0.548511938237031,	0.548135293118453,	0.547759365533147,	0.547384148138627,	0.547009633692591,	0.546635815051095,	0.54626268516681,	0.545890237087279,	0.54551846395322,	0.545147358991789,	0.5447769155416,	0.54440712700146,	0.544037986866912,	0.543669488717483,	0.543301626224108,	0.542934393118288,	0.542567783274599,	0.542201790572777,	0.541836409000926,	0.541471632609927,	0.541107455569497,	0.54074387209592,	0.540380876439056,	0.54001846299497,	0.539656626169489,	0.539295360473212,	0.538934660489081,	0.538574520799644,	0.538214936170375,	0.537855901326209,	0.53749741110073,	0.537139460413584,	0.536782044188622,	0.536425157485237,	0.536068795321596,	0.535712952866797,	0.535357625339514,	0.535002807932449,	0.53464849599529,	0.534294684836635,	0.533941369963195,	0.533588546776208,	0.533236210813243,	0.532884357679934,	0.532532982962028,	0.532182082334433,	0.531831651556074,	0.531481686396139,	0.531132182662448,	0.530783136239154,	0.530434543048508,	0.530086399042481,	0.529738700231291,	0.529391442656908,	0.52904462245527,	0.52869823574043,	0.528352278726561,	0.528006747611412,	0.527661638531511,	0.527316948127628,	0.526972672411958,	0.526628808102363,	0.52628535139709,	0.525942298548372,	0.525599646628993,	0.525257391826855,	0.524915530691932,	0.524574059891547,	0.52423297609254,	0.523892275982721,	0.523551956283599,	0.523212013750727,	0.522872445173442,	0.522533247374458,	0.522194417209414,	0.521855951566416,	0.521517847365596,	0.521180101558659,	0.520842711128453,	0.520505673088536,	0.520168984482756,	0.519832642384835,	0.519496643897962,	0.519160986154393,	0.518825666315053,	0.518490681569152,	0.518156029133797,	0.517821706253626,	0.517487710200428,	0.517154038272787,	0.51682068779572,	0.51648765612033,	0.516154940623452,	0.515822538707319,	0.515490447799224,	0.51515866535119,	0.514827188839644,	0.5144960157651,	0.514165143651842,	0.513834570047615,	0.513504292523319,	0.513174308672709,	0.5128446161121,	0.512515212480077,	0.5121860954372,	0.51185726266573,	0.51152871186934,	0.51120044077293,	0.510872447122627,	0.510544728674665,	0.510217283260449,	0.509890108586377,	0.509563202604663,	0.509236563090964,	0.508910187916088,	0.508584074961097,	0.508258222110556,	0.507932627350058,	0.507607288607235,	0.50728220375631,	0.506957370902318,	0.506632787936135,	0.506308452886638,	0.505984363851817,	0.505660518767163,	0.505336915815296,	0.505013553001752,	0.504690428425993,	0.50436754020756,	0.504044886485251,	0.503722465379402,	0.503400275146095,	0.50307831380283,	0.502756579696617,	0.502435070914173,	0.502113785712436,	0.501792722343284,	0.501471879029121,	0.501151254110007,	0.500830845754136,	0.50051065235352,	0.500190672105032,	0.499870903488885,	0.499551344637181,	0.499231994065218,	0.498912850090431,	0.498593911057023,	0.49827517534908,	0.497956641393929,	0.497638307592075,	0.497320172390868,	0.497002234142623,	0.496684491379496,	0.496366942570767,	0.496049586143279,	0.495732420563645,	0.495415444392645,	0.495098656127211,	0.494782054254426,	0.494465637302582,	0.494149403832132,	0.493833352407298,	0.493517481563791,	0.493201789907419,	0.492886275980506,	0.492570938409373,	0.492255775785807,	0.491940786736754,	0.491625969862435,	0.491311323847218,	0.490996847351177,	0.490682538919204,	0.49036839727835,	0.490054421165688,	0.489740609128333,	0.489426960050496,	0.489113472415316,	0.48880014517509,	0.488486976848825,	0.488173966245287,	0.487861112098389,	0.487548413155343,	0.487235868172249,	0.486923475913778,	0.486611235153033,	0.486299144671451,	0.485987203258706,	0.485675409712615,	0.485363762839048,	0.485052261451832,	0.48474090437267,	0.484429690431039,	0.484118618464116,	0.483807687316681,	0.483496895841033,	0.483186242896906,	0.482875727351333,	0.482565348078644,	0.482255103960374,	0.481944993885166,	0.481635016748684,	0.481325171453537,	0.481015456909199,	0.480705872031931,	0.480396415744703,	0.480087086977119,	0.479777884665342,	0.479468807752018,	0.479159855186203,	0.478851025936817,	0.478542318942281,	0.478233733176577,	0.4779252676169,	0.477616921243581,	0.477308693042667,	0.477000582006079,	0.476692587131583,	0.476384707422721,	0.476076941888747,	0.475769289544562,	0.475461749410648,	0.475154320513002,	0.474847001883076,	0.474539792557709,	0.474232691579065,	0.473925697994575,	0.47361881085687,	0.473312029223728,	0.473005352158009,	0.472698778727601,	0.472392308005371,	0.472085939069128,	0.471779671001597,	0.471473502890425,	0.471167433828033,	0.470861462910275,	0.470555589233065,	0.47024981190279,	0.469944130047852,	0.469638542783065,	0.469333049196514,	0.469027648420998,	0.468722339594328,	0.46841712188916,	0.468111994351163,	0.46780695621336,	0.467502006536198,	0.467197144562893,	0.466892369304976,	0.466587680089126,	0.466283075933118,	0.465978556087905,	0.465674119703099,	0.465369765938534,	0.465065493957738,	0.464761303037676,	0.464457192111782,	0.464153160760792,	0.463849207694941,	0.463545332576999,	0.463241534250143,	0.462937812099013,	0.462634165286128,	0.462330592967336,	0.462027094463452,	0.461723668850719,	0.461420315431563,	0.461117033483034,	0.460813821955485,	0.460510680508517,	0.460207607995992,	0.459904603832758,	0.459601667154779,	0.459298797261369,	0.458995993449887,	0.4586932548218,	0.45839058071478,	0.458087970334978,	0.457785422950773,	0.457482937849662,	0.457180514225224,	0.456878151351743,	0.456575848581145,	0.456273604987858,	0.455971420007247,	0.455669292866785,	0.455367222740302,	0.455065209075244,	0.454763250929644,	0.454461347777173,	0.454159498808903,	0.453857703286892,	0.453555960553728,	0.453254269801298,	0.452952630405559,	0.4526510417054,	0.452349502783557,	0.452048013080266,	0.45174657189268,	0.451445178570679,	0.45114383228926,	0.450842532350345,	0.450541278137239,	0.450240068892356,	0.449938903981608,	0.449637782622459,	0.449336704247428,	0.44903566806391,	0.448734673404283,	0.448433719597252,	0.44813280594355,	0.447831931774907,	0.447531096390044,	0.447230299127363,	0.446929539274822,	0.446628816180969,	0.446328129158048,	0.446027477529052,	0.445726860617968,	0.445426277749871,	0.445125728250898,	0.444825211448212,	0.444524726669965,	0.444224273245267,	0.443923850504148,	0.443623457777523,	0.443323094397161,	0.443022759695643,	0.442722453006337,	0.442422173663352,	0.442121921001514,	0.441821694356321,	0.441521493063918,	0.441221316461054,	0.440921163885052,	0.440621034673771,	0.440320928165576,	0.440020843699297,	0.439720780614197,	0.439420738249938,	0.439120715946545,	0.438820713044369,	0.438520728884057,	0.438220762806511,	0.437920814152856,	0.437620882264404,	0.43732096648262,	0.437021066149084,	0.436721180605457,	0.436421309193445,	0.436121451254767,	0.43582160613111,	0.435521773164106,	0.435221951695283,	0.43492214106604,	0.434622340617763,	0.434322549690155,	0.43402276762702,	0.433722993766509,	0.433423227448763,	0.433123468014134,	0.432823714802121,	0.432523967152108,	0.432224224401507,	0.431924485890281,	0.431624750953079,	0.431325018930044,	0.431025289154177,	0.430725560964094,	0.43042583369471,	0.430126106678174,	0.429826379248266,	0.42952665073933,	0.429226920482744,	0.428927187806395,	0.428627452043877,	0.428327712523955,	0.428027968574729,	0.427728219522707,	0.427428464690329,	0.427128703409812,	0.426828934997685,	0.426529158781296,	0.426229374079177,	0.425929580212375,	0.42562977649958,	0.425329962254522,	0.425030136797579,	0.424730299442719,	0.424430449501528,	0.42413058628292,	0.423830709100046,	0.423530817261442,	0.423230910070433,	0.422930986831114,	0.422631046851518,	0.422331089430848,	0.422031113864442,	0.421731119451332,	0.421431105490164,	0.4211310712711,	0.420831016086586,	0.420530939223448,	0.420230839973704,	0.419930717619504,	0.419630571442299,	0.419330400724947,	0.419030204742083,	0.418729982772684,	0.418429734087894,	0.418129457960157,	0.417829153655104,	0.417528820443371,	0.417228457577874,	0.416928064332816,	0.416627639955097,	0.416327183702502,	0.416026694827427,	0.415726172578341,	0.415425616200941,	0.415125024944362,	0.414824398015603,	0.414523734698122,	0.414223034202923,	0.41392229576429,	0.41362151862418,	0.41332070195322,	0.413019845030817,	0.412718947041283,	0.412418007208583,	0.412117024739612,	0.4118159988346,	0.411514928708015,	0.411213813534107,	0.410912652533577,	0.410611444883173,	0.410310189772159,	0.410008886379431,	0.409707533887796,	0.409406131465105,	0.409104678282024,	0.408803173504147,	0.408501616292908,	0.4082000058043,	0.407898341184964,	0.407596621587185,	0.407294846150699,	0.406993014012949,	0.406691124301818,	0.406389176145364,	0.406087168671261,	0.405785100988039,	0.405482972212758,	0.4051807814517,	0.404878527799872,	0.404576210357416,	0.404273828212778,	0.403971380449219,	0.403668866145016,	0.403366284372361,	0.403063634197469,	0.402760914680489,	0.402458124875418,	0.402155263829993,	0.401852330585603,	0.40154932417718,	0.401246243633102,	0.400943087975087,	0.400639856218089,	0.400336547370195,	0.40003316043251,	0.399729694399054,	0.399426148256646,	0.399122520984796,	0.398818811555582,	0.398515018933545,	0.39821114207556,	0.397907179930722,	0.397603131440222,	0.397298995537224,	0.396994771146737,	0.396690457185492,	0.396386052561805,	0.396081556175451,	0.395776966917527,	0.395472283670317,	0.395167505307151,	0.394862630692269,	0.394557658680674,	0.394252588117985,	0.393947417840295,	0.393642146674018,	0.393336773435732,	0.39303129693203,	0.392725715959358,	0.392420029303857,	0.392114235741196,	0.391808334036409,	0.391502322943724,	0.391196201206394,	0.390889967556515,	0.390583620714858,	0.390277159390677,	0.389970582281534,	0.389663888073104,	0.389357075438991,	0.389050143040526,	0.388743089526146,	0.388435913533783,	0.38812861368469,	0.387821188589064,	0.387513636845599,	0.387205957036575,	0.386898147732427,	0.38659020748747,	0.38628213484468,	0.385973928330107,	0.385665586457517,	0.385357107723266,	0.385048490610716,	0.384739733586389,	0.384430835101166,	0.384121793590551,	0.383812607482504,	0.383503275180435,	0.383193795046537,	0.382884165464183,	0.382574384786008,	0.382264451347001,	0.38195436346227,	0.381644119431125,	0.381333717532974,	0.381023156028397,	0.380712433156762,	0.380401547146341,	0.380090496197754,	0.379779278491939,	0.379467892185366,	0.379156335423623,	0.378844606323353,	0.378532702985202,	0.378220623484666,	0.377908365875054,	0.377595928187238,	0.377283308429672,	0.376970504587258,	0.37665751461801,	0.376344336459683,	0.376030968022066,	0.37571740718969,	0.375403651823667,	0.375089699755973,	0.374775548795217,	0.37446119671689,	0.374146641277617,	0.373831880195763,	0.373516911168818,	0.373201731859205,	0.372886339904367,	0.372570732908035,	0.37225490844483,	0.371938864056513,	0.371622597253624,	0.371306105511962,	0.370989386275156,	0.370672436954306,	0.370355254924226,	0.370037837523253,	0.369720182052986,	0.369402285782669,	0.369084145938783,	0.368765759713298,	0.36844712425893,	0.368128236682108,	0.367809094058769,	0.367489693414968,	0.367170031740227,	0.366850105975975,	0.366529913022822,	0.366209449735527,	0.365888712923699,	0.365567699347921,	0.365246405721821,	0.364924828712867,	0.364602964934851,	0.364280810955003,	0.36395836335149,	0.36363561853465,	0.36331257289353,	0.36298922277358,	0.362665564470728,	0.362341594218184,	0.362017308191243,	0.36169270250876,	0.361367773222024,	0.361042516321858,	0.360716927735745,	0.360391003322067,	0.360064738874866,	0.359738130118209,	0.359411172702929,	0.359083862211693,	0.358756194144921,	0.358428163941993,	0.358099766957332,	0.357770998459491,	0.357441853645603,	0.357112327623728,	0.356782415418071,	0.356452112148187,	0.356121412709278,	0.355790311784204,	0.355458803982421,	0.355126883837578,	0.354794545802861,	0.354461784229405,	0.354128593379837,	0.353794967404612,	0.353460900359167,	0.353126386177485,	0.352791418700071,	0.352455991661628,	0.352120098562174,	0.351783732776785,	0.351446887874355,	0.351109555842677,	0.350771723528572,	0.350433384985556,	0.350094535307452,	0.349755168622186,	0.349415278357306,	0.349074857441516,	0.348733898430334,	0.348392393583121,	0.348050334909478,	0.347707714223539,	0.347364523054849,	0.347020752800759,	0.346676394646465,	0.346331439575221,	0.345985878368804,	0.34563970160393,	0.345292899647368,	0.344945462650391,	0.344597380542708,	0.344248643025995,	0.343899239567061,	0.343549159390678,	0.343198391472099,	0.342846924529252,	0.342494747014612,	0.342141847106739,	0.341788212701468,	0.341433831402751,	0.341078690513105,	0.340722777023683,	0.340366077603923,	0.340008578590764,	0.339650265977414,	0.339291125401628,	0.338931142133497,	0.338570301062696,	0.338208586685184,	0.337845983089313,	0.33748247394132,	0.337118042470175,	0.336752671451731,	0.336386343192164,	0.33601903951064,	0.335650741721183,	0.335281430613681,	0.334911086434009,	0.334539688863181,	0.334167216995513,	0.333793649315707,	0.333418963674982,	0.333043137266985,	0.332666146596966,	0.332287967458389,	0.331908574902245,	0.331527943206254,	0.331146045842424,	0.33076285544293,	0.330378343764169,	0.329992481648869,	0.329605238986137,	0.329216584669287,	0.328826486551322,	0.328434911397894,	0.32804182483758,	0.327647191309285,	0.327250974006559,	0.326853134818636,	0.326453634267923,	0.326052431443717,	0.325649483931844,	0.325244747739933,	0.324838177217988,	0.324429724973902,	0.324019341783516,	0.323606976494804,	0.323192575925713];
eff=interp1(fc_pwr_map,fc_eff_map,P_fc);

== matlab function FCEvReferenceApplication/Subsystem/MATLAB Function ==
  data: mot_spd output; veh_spd input; mot_trq output; veh_acc input
function [mot_spd,mot_trq] = fcn(veh_spd,veh_acc)
veh_whl_radius = 0.327;
veh_mass = 1500;
veh_rrc  = 0.015;
veh_air_density = 1.2;
veh_FA = 2.27;
veh_CD = 0.28;
veh_gravity = 9.81;
veh_fd_ratio = 7.94;

w_whl = veh_spd ./ veh_whl_radius;
F_roll = (veh_spd > 0) .* veh_mass .* veh_gravity .* veh_rrc;
F_drag = 0.5 .* veh_air_density .* veh_FA .* veh_CD .* (veh_spd.^2);
F_acc = veh_mass .* veh_acc;
T_whl = veh_whl_radius .* (F_acc + F_roll + F_drag);
mot_t = T_whl./veh_fd_ratio;
mot_trq = mot_t;
mot_spd = w_whl.*veh_fd_ratio;
